simulink model "SIMULINK_Trim"  (R2020a)
settings: Solver=VariableStepAuto  StartTime=0.0  StopTime=10.0  RelTol=1e-3
settings Model: Creator=CepaTech  LastModifiedBy=CepaTech

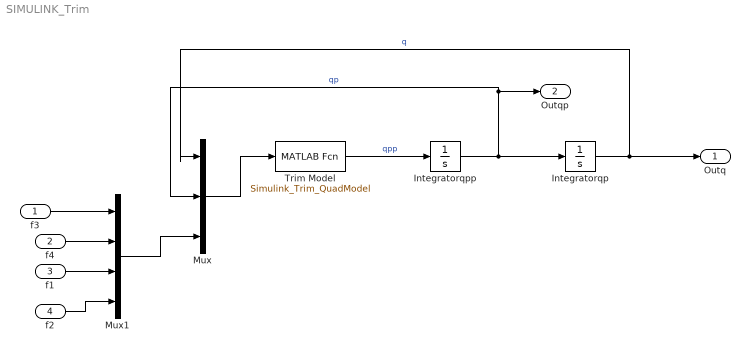
== system SIMULINK_Trim ==
  f3 : Inport
  f4 : Inport  Port=2
  f1 : Inport  Port=3
  f2 : Inport  Port=4
  Integratorqp : Integrator  InitialCondition=[0 0 0 0 0 0]
  Integratorqpp : Integrator  InitialCondition=[0 0 0 0 0 0]
  Mux : Mux  Inputs=3
  Mux1 : Mux
  Trim Model : MATLABFcn  MATLABFcn=Simulink_Trim_QuadModel
  Outq : Outport
  Outqp : Outport  Port=2
  wires:
  Trim Model/1 -> Integratorqpp/1  "qpp"
  Integratorqpp/1 -> Outqp/1, Mux/2, Integratorqp/1  "qp"
  Mux/1 -> Trim Model/1
  f4/1 -> Mux1/2
  Mux1/1 -> Mux/3
  f3/1 -> Mux1/1
  f1/1 -> Mux1/3
  f2/1 -> Mux1/4
  Integratorqp/1 -> Mux/1, Outq/1  "q"
